simulink library "ddr4_behavioral_mdl"  (R2019b)
settings: Solver=VariableStepAuto  StartTime=0.0  StopTime=10.0  RelTol=1e-3
libraries: hdlsllib x7, simulink x4, AXIDMALib x1
settings Model: Creator=darenlee  LastModifiedBy=ajtro

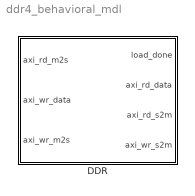
== system ddr4_behavioral_mdl ==
  DDR : Subsystem  mask{DDR3_DEPTH=1024, WR_RD_DATAWIDTH=128, INIT_DDR3=on, INIT_ADDR=0, INIT_DATA=fi(zeros(1,1024),0,128,0), OutDataTypeStr=fixdt(0,128,0), READY_DUTY_CYL=1, toggle=off}
      mask prompts: DDR3_DEPTH "DDR DEPTH"; WR_RD_DATAWIDTH "DDR Data Width"; INIT_DDR3 "Initialize DDR"; INIT_ADDR "DDR Initial Address"; INIT_DATA "DDR Initialization data"; OutDataTypeStr "Simulink:blkprm_prompts:UNIFIEDDATATYPE"; READY_DUTY_CYL "READY Duty Cycle"; toggle "Read Valid Toggling"
      mask help: DDR Simulation model
      mask init:
      | if(DDR3_DEPTH<=1)
      |     error('DDR size should be greater than 1' )  
      | end
      | 
      | if(READY_DUTY_CYL>1)
      |   error('should be less than 1' )  
      | end
      |    
      | 
      | %%Initialization Value
      | if(INIT_DDR3==true)
      |     if(isempty(INIT_ADDR))
      |      error('Enter Initial address' )  
      |     end   
      | end
      mask TypeOptions WR_RD_DATAWIDTH: 32 | 64 | 128
      mask Callback INIT_DDR3:
      | % Get the mask parameter values. This is a cell
      | %   array of character vectors.
      | maskStr = get_param(gcb,'INIT_DDR3');
      | 
      | % The pop-up menu is the first mask parameter.
      | %   Check the value selected in the pop-up
      | if strcmp(maskStr,'on')
      | 
      |     % Set the visibility of both parameters on when
      |     %   User-defined is selected in the pop-up.
      | 
      |     set_param(gcb,'MaskEnables',{'on','on','on','on','on','on','on','on'});
      | 
      | else
      | 
      |     % Turn off the visibility of the Value field
      |     %   when User-defined is not selected.
      | 
      |     set_param(gcb,'MaskEnables',{'on','on','on','off','off','on','on','on'});
      | 
      |     % Set the character vector in the Values field equal to the
      |     % character vector selected in the Gain pop-up menu.
      | 
      |     %maskStr{2}=maskStr{1};
      | 
      | end
      mask TypeOptions OutDataTypeStr: axi_wr_data/OutDataTypeStr | axi_rd_data/OutDataTypeStr
      mask DialogControl DescGroupVar Prompt: DDR
      mask DialogControl DDR3_INIT Prompt: DDR Initialization
      mask DialogControl PARAM_GROUP Prompt: DDR Initialization Parameters
      mask DialogControl OutDataTypeStr Prompt: Data type:
      mask DialogControl READY_DUTY_CYL Tooltip: between 0 to 1

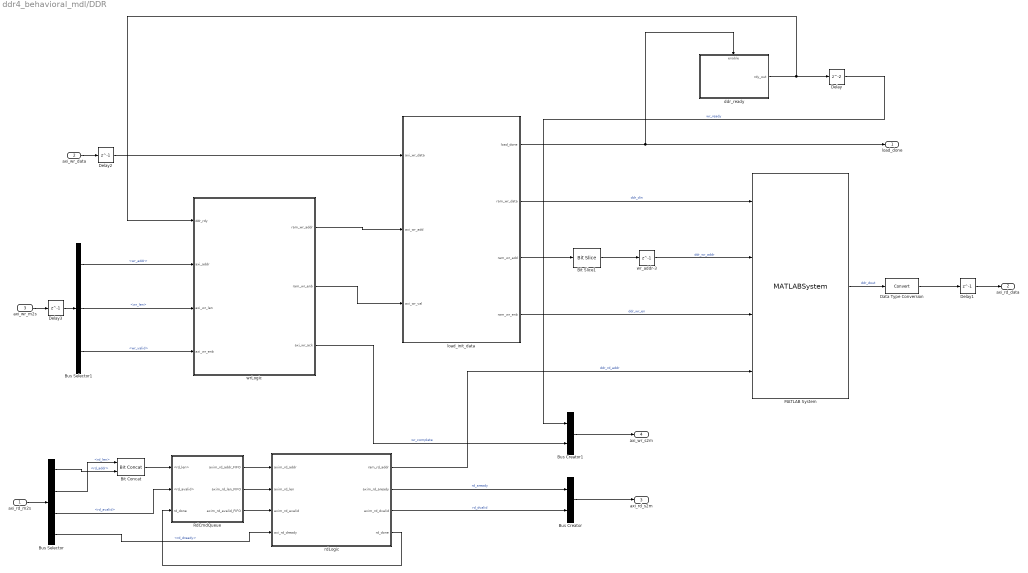
== system ddr4_behavioral_mdl/DDR ==
  axi_rd_m2s : Inport
  axi_wr_data : Inport  Port=2  OutDataTypeStr=fixdt(0,128,0)
  axi_wr_m2s : Inport  Port=3
  Bit Concat : hdlsllib/Logic and Bit Operations/Bit Concat  numInputs=2
      settings: SourceProductName=Simulink
  Bit Slice1 : hdlsllib/Logic and Bit Operations/Bit Slice  lidx=15  ridx=0
  Bus Creator : BusCreator  Inputs=2
  Bus Creator1 : BusCreator  Inputs=2
  Bus Selector : BusSelector  OutputSignals=rd_addr,rd_len,rd_avalid,rd_dready
  Bus Selector1 : BusSelector  OutputSignals=wr_addr,wr_len,wr_valid
  Data Type Conversion : DataTypeConversion
  Delay : Delay
  Delay1 : Delay  DelayLength=1
  Delay2 : Delay  DelayLength=1
  Delay3 : Delay  DelayLength=1
  MATLAB System : MATLABSystem  System=hdl.RAM  RAMType=Simple dual port  WriteOutputValue=New data  RAMInitialValue=0  SimulateUsing=Code generation
      mask Type: hdl.RAM
      mask Display:
      | disp(['Simple' char(10) 'Dual Port' char(10) 'RAM']);
      | port_label('input',1,'din');
      | port_label('input',2,'wr_addr');
      | port_label('input',3,'wr_en');
      | port_label('input',4,'rd_addr');
      | port_label('output',1,'rd_dout');
  RdCmdQueue : Subsystem
  ddr_ready : Subsystem
  load_init_data : MATLAB Function  TreatAsAtomicUnit=on
  rdLogic : Subsystem
  wrLogic : Subsystem
  wr_addr-3 : Delay  DelayLength=1
  load_done : Outport  VectorParamsAs1DForOutWhenUnconnected=off
  axi_rd_data : Outport  Port=2  OutDataTypeStr=fixdt(0,128,0)  VectorParamsAs1DForOutWhenUnconnected=off
  axi_rd_s2m : Outport  Port=3  VectorParamsAs1DForOutWhenUnconnected=off
  axi_wr_s2m : Outport  Port=4  VectorParamsAs1DForOutWhenUnconnected=off
  wires:
  Bit Slice1/1 -> wr_addr-3/1
  Delay1/1 -> axi_rd_data/1
  load_init_data/4(ram_wr_enb) -> MATLAB System/3  "ddr_wr_en"
  load_init_data/3(ram_wr_add) -> Bit Slice1/1
  load_init_data/1(load_done) -> ddr_ready/Enable, load_done/1
  MATLAB System/1 -> Data Type Conversion/1  "ddr_dout"
  rdLogic/1(ram_rd_addr) -> MATLAB System/4  "ddr_rd_addr"
  wrLogic/1(ram_wr_addr) -> load_init_data/2(axi_wr_add)
  wrLogic/2(ram_wr_enb) -> load_init_data/3(axi_wr_val)
  wr_addr-3/1 -> MATLAB System/2  "ddr_wr_addr"
  Bus Selector/1 -> Bit Concat/2  "<rd_addr>"
  Bus Selector/4 -> rdLogic/4(axi_rd_dready)  "<rd_dready>"
  axi_rd_m2s/1 -> Bus Selector/1
  Bus Selector1/1 -> wrLogic/2(axi_addr)  "<wr_addr>"
  axi_wr_m2s/1 -> Delay3/1
  Bus Selector1/3 -> wrLogic/4(axi_wr_enb)  "<wr_valid>"
  Bus Selector1/2 -> wrLogic/3(axi_wr_len)  "<wr_len>"
  rdLogic/2(axim_rd_aready) -> Bus Creator/1  "rd_aready"
  Bus Creator/1 -> axi_rd_s2m/1
  rdLogic/3(axim_rd_dvalid) -> Bus Creator/2  "rd_dvalid"
  ddr_ready/1(rdy_out) -> Delay/1, wrLogic/1(ddr_rdy)
  Bus Creator1/1 -> axi_wr_s2m/1
  wrLogic/3(axi_wr_ack) -> Bus Creator1/2  "wr_complete"
  Delay/1 -> Bus Creator1/1  "wr_ready"
  load_init_data/2(ram_wr_data) -> MATLAB System/1  "ddr_din"
  axi_wr_data/1 -> Delay2/1
  Delay2/1 -> load_init_data/1(axi_wr_data)
  Delay3/1 -> Bus Selector1/1
  Data Type Conversion/1 -> Delay1/1
  Bus Selector/2 -> Bit Concat/1  "<rd_len>"
  Bus Selector/3 -> RdCmdQueue/2(<rd_avalid>)  "<rd_avalid>"
  RdCmdQueue/2(axim_rd_len_FIFO) -> rdLogic/2(axim_rd_len)
  RdCmdQueue/3(axim_rd_avalid_FIFO) -> rdLogic/3(axim_rd_avalid)
  rdLogic/4(rd_done) -> RdCmdQueue/3(rd_done)
  Bit Concat/1 -> RdCmdQueue/1(<rd_len>)
  RdCmdQueue/1(axim_rd_addr_FIFO) -> rdLogic/1(axim_rd_addr)

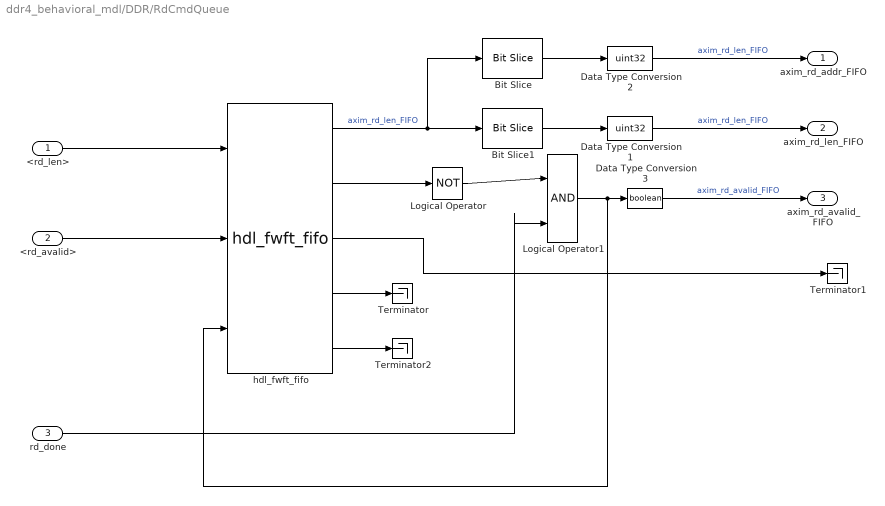
== system ddr4_behavioral_mdl/DDR/RdCmdQueue ==
  <rd_len> : Inport
  <rd_avalid> : Inport  Port=2
  rd_done : Inport  Port=3
  Bit Slice : hdlsllib/Logic and Bit Operations/Bit Slice  lidx=31  ridx=0
      settings: SourceProductName=Simulink  SourceProductBaseCode=SL
  Bit Slice1 : hdlsllib/Logic and Bit Operations/Bit Slice  lidx=63  ridx=32
      settings: SourceProductName=Simulink  SourceProductBaseCode=SL
  Data Type Conversion1 : DataTypeConversion  OutDataTypeStr=uint32
  Data Type Conversion2 : DataTypeConversion  OutDataTypeStr=uint32
  Data Type Conversion3 : DataTypeConversion  OutDataTypeStr=boolean
  Logical Operator : Logic  Operator=NOT  IconShape=distinctive  AllPortsSameDT=off  OutDataTypeStr=boolean
  Logical Operator1 : Logic  IconShape=distinctive  AllPortsSameDT=off  OutDataTypeStr=boolean
  Terminator : Terminator
  Terminator1 : Terminator
  Terminator2 : Terminator
  hdl_fwft_fifo : AXIDMALib/Hardware/hdl_fwft_fifo  FIFO_DEPTH=1*1024  AFULL_THRESH=ceil(1*1024*0.1)
  axim_rd_addr_FIFO : Outport  VectorParamsAs1DForOutWhenUnconnected=off
  axim_rd_len_FIFO : Outport  Port=2
  axim_rd_avalid_FIFO : Outport  Port=3
  wires:
  hdl_fwft_fifo/3 -> Terminator1/1
  Logical Operator1/1 -> hdl_fwft_fifo/3, Data Type Conversion3/1
  hdl_fwft_fifo/4 -> Terminator/1
  hdl_fwft_fifo/2 -> Logical Operator/1
  <rd_avalid>/1 -> hdl_fwft_fifo/2
  hdl_fwft_fifo/5 -> Terminator2/1
  Logical Operator/1 -> Logical Operator1/1
  Data Type Conversion3/1 -> axim_rd_avalid_FIFO/1  "axim_rd_avalid_FIFO"
  hdl_fwft_fifo/1 -> Bit Slice1/1, Bit Slice/1  "axim_rd_len_FIFO"
  <rd_len>/1 -> hdl_fwft_fifo/1
  rd_done/1 -> Logical Operator1/2
  Data Type Conversion1/1 -> axim_rd_len_FIFO/1  "axim_rd_len_FIFO"
  Bit Slice1/1 -> Data Type Conversion1/1
  Bit Slice/1 -> Data Type Conversion2/1
  Data Type Conversion2/1 -> axim_rd_addr_FIFO/1  "axim_rd_len_FIFO"

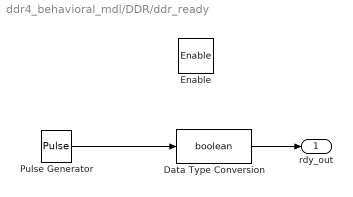
== system ddr4_behavioral_mdl/DDR/ddr_ready ==
  Enable : EnablePort
  Data Type Conversion : DataTypeConversion  OutDataTypeStr=boolean
  Pulse Generator : DiscretePulseGenerator  Period=1000  PulseWidth=1000 * READY_DUTY_CYL  SampleTime=-1
  rdy_out : Outport  VectorParamsAs1DForOutWhenUnconnected=off
  wires:
  Pulse Generator/1 -> Data Type Conversion/1
  Data Type Conversion/1 -> rdy_out/1

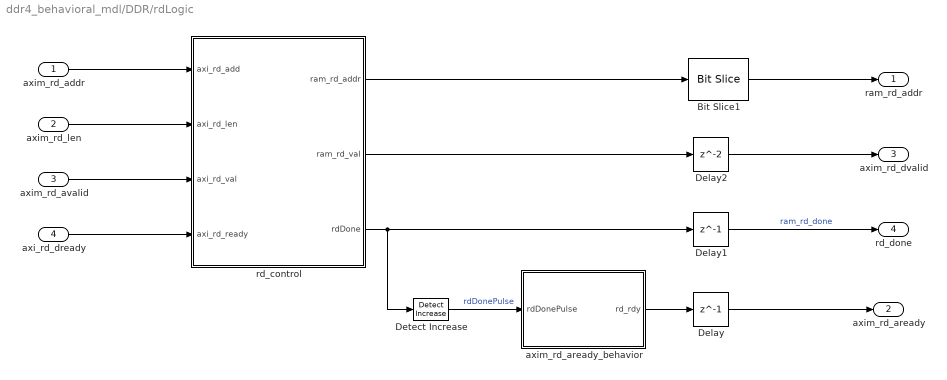
== system ddr4_behavioral_mdl/DDR/rdLogic ==
  axim_rd_addr : Inport
  axim_rd_len : Inport  Port=2
  axim_rd_avalid : Inport  Port=3
  axi_rd_dready : Inport  Port=4
  Bit Slice1 : hdlsllib/Logic and Bit Operations/Bit Slice  lidx=15  ridx=0
  Delay : Delay  DelayLength=1
  Delay1 : Delay  DelayLength=1
  Delay2 : Delay
  Detect Increase : simulink/Logic and Bit Operations/Detect Increase  vinit=0.0  OutDataTypeStr=boolean
  axim_rd_aready_behavior : MATLAB Function  TreatAsAtomicUnit=on
  rd_control : MATLAB Function  TreatAsAtomicUnit=on
  ram_rd_addr : Outport  VectorParamsAs1DForOutWhenUnconnected=off
  axim_rd_aready : Outport  Port=2  VectorParamsAs1DForOutWhenUnconnected=off
  axim_rd_dvalid : Outport  Port=3  VectorParamsAs1DForOutWhenUnconnected=off
  rd_done : Outport  Port=4  VectorParamsAs1DForOutWhenUnconnected=off
  wires:
  Delay/1 -> axim_rd_aready/1
  Detect Increase/1 -> axim_rd_aready_behavior/1(rdDonePulse)  "rdDonePulse"
  rd_control/3(rdDone) -> Delay1/1, Detect Increase/1
  axim_rd_aready_behavior/1(rd_rdy) -> Delay/1
  axim_rd_addr/1 -> rd_control/1(axi_rd_add)
  rd_control/1(ram_rd_addr) -> Bit Slice1/1
  axim_rd_avalid/1 -> rd_control/3(axi_rd_val)
  Bit Slice1/1 -> ram_rd_addr/1
  axi_rd_dready/1 -> rd_control/4(axi_rd_ready)
  Delay2/1 -> axim_rd_dvalid/1
  axim_rd_len/1 -> rd_control/2(axi_rd_len)
  rd_control/2(ram_rd_val) -> Delay2/1
  Delay1/1 -> rd_done/1  "ram_rd_done"

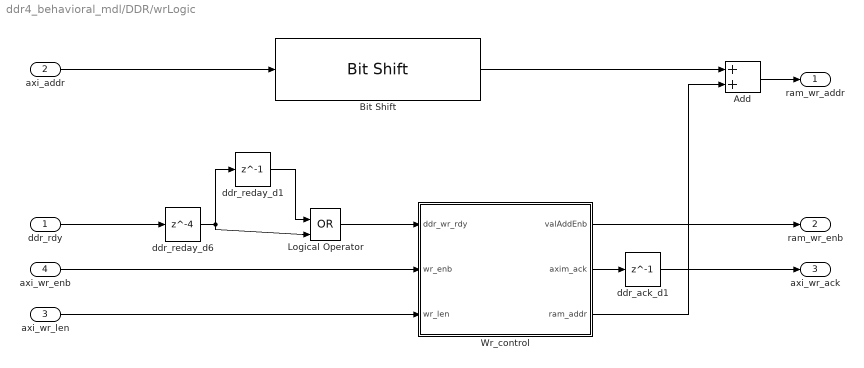
== system ddr4_behavioral_mdl/DDR/wrLogic ==
  ddr_rdy : Inport
  axi_addr : Inport  Port=2
  axi_wr_len : Inport  Port=3
  axi_wr_enb : Inport  Port=4
  Add : Sum  AccumDataTypeStr=uint32
  Bit Shift : hdlsllib/Logic and Bit Operations/Bit Shift  mode=Shift Right Arithmetic  N=log2(WR_RD_DATAWIDTH/8)
      settings: SourceProductName=HDL Coder  SourceProductBaseCode=HD
  Logical Operator : Logic  Operator=OR  IconShape=distinctive  AllPortsSameDT=off  OutDataTypeStr=boolean
  Wr_control : Subsystem
  ddr_ack_d1 : Delay  DelayLength=1
  ddr_reday_d1 : Delay  DelayLength=1
  ddr_reday_d6 : Delay  DelayLength=4
  ram_wr_addr : Outport  VectorParamsAs1DForOutWhenUnconnected=off
  ram_wr_enb : Outport  Port=2  VectorParamsAs1DForOutWhenUnconnected=off
  axi_wr_ack : Outport  Port=3  VectorParamsAs1DForOutWhenUnconnected=off
  wires:
  Wr_control/1(valAddEnb) -> ram_wr_enb/1
  axi_wr_len/1 -> Wr_control/3(wr_len)
  ddr_rdy/1 -> ddr_reday_d6/1
  axi_wr_enb/1 -> Wr_control/2(wr_enb)
  Wr_control/2(axim_ack) -> ddr_ack_d1/1
  Add/1 -> ram_wr_addr/1
  Wr_control/3(ram_addr) -> Add/2
  ddr_reday_d6/1 -> ddr_reday_d1/1, Logical Operator/2
  ddr_ack_d1/1 -> axi_wr_ack/1
  axi_addr/1 -> Bit Shift/1
  ddr_reday_d1/1 -> Logical Operator/1
  Logical Operator/1 -> Wr_control/1(ddr_wr_rdy)
  Bit Shift/1 -> Add/1

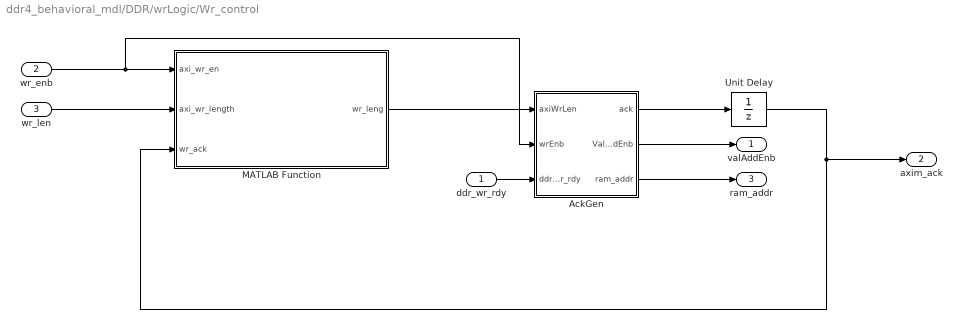
== system ddr4_behavioral_mdl/DDR/wrLogic/Wr_control ==
  ddr_wr_rdy : Inport
  wr_enb : Inport  Port=2
  wr_len : Inport  Port=3
  AckGen : Subsystem
  MATLAB Function : MATLAB Function  TreatAsAtomicUnit=on
  Unit Delay : UnitDelay  SampleTime=-1  HasFrameUpgradeWarning=on
  valAddEnb : Outport  VectorParamsAs1DForOutWhenUnconnected=off
  axim_ack : Outport  Port=2  VectorParamsAs1DForOutWhenUnconnected=off
  ram_addr : Outport  Port=3  VectorParamsAs1DForOutWhenUnconnected=off
  wires:
  wr_enb/1 -> AckGen/2(wrEnb), MATLAB Function/1(axi_wr_en)
  AckGen/2(ValAddEnb) -> valAddEnb/1
  wr_len/1 -> MATLAB Function/2(axi_wr_length)
  AckGen/1(ack) -> Unit Delay/1
  MATLAB Function/1(wr_leng) -> AckGen/1(axiWrLen)
  Unit Delay/1 -> axim_ack/1, MATLAB Function/3(wr_ack)
  AckGen/3(ram_addr) -> ram_addr/1
  ddr_wr_rdy/1 -> AckGen/3(ddr_wr_rdy)

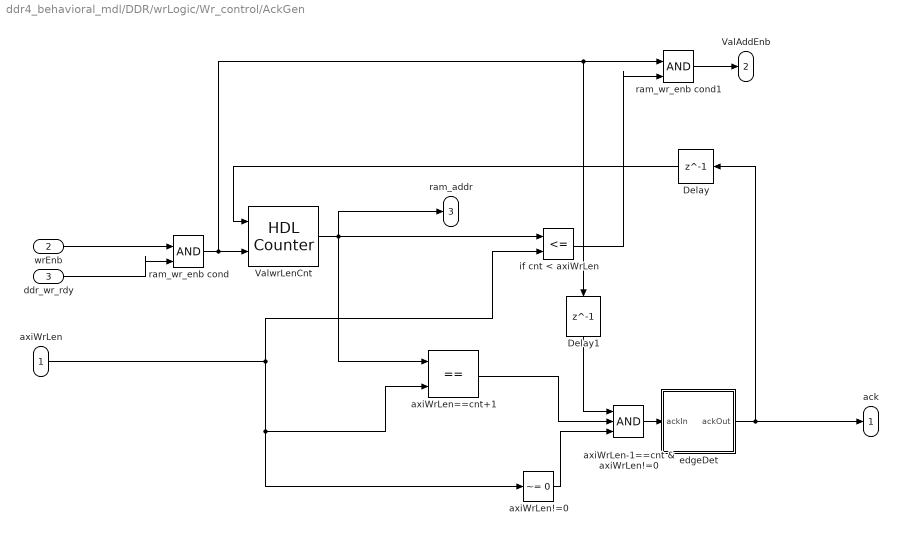
== system ddr4_behavioral_mdl/DDR/wrLogic/Wr_control/AckGen ==
  axiWrLen : Inport
  wrEnb : Inport  Port=2
  ddr_wr_rdy : Inport  Port=3
  Delay : Delay  DelayLength=1
  Delay1 : Delay  DelayLength=1
  ValwrLenCnt : hdlsllib/Sources/HDL Counter  CountType=Free running  CountInit=0  CountStep=1  CountMax=DDR3_DEPTH  CountFromType=Initial value  CountFrom=0  CountResetPort=on  CountLoadPort=off  CountEnbPort=on  CountDirPort=off  CountDataType=Unsigned  CountWordLen=32  CountFracLen=0  CountSampTime=1
      settings: SourceProductBaseCode=HD
  axiWrLen!=0 : simulink/Logic and Bit Operations/Compare To Constant  relop=~=  const=0  OutDataTypeStr=boolean
  "axiWrLen-1==cnt & axiWrLen!=0 " : Logic  Inputs=3  IconShape=distinctive  AllPortsSameDT=off  OutDataTypeStr=boolean
  axiWrLen==cnt+1 : RelationalOperator  Operator===  OutDataTypeStr=boolean  RndMeth=Nearest
  edgeDet : Subsystem
  if cnt < axiWrLen : RelationalOperator  Operator=<=  OutDataTypeStr=boolean  RndMeth=Nearest
  ram_wr_enb cond : Logic  IconShape=distinctive  AllPortsSameDT=off  OutDataTypeStr=boolean
  ram_wr_enb cond1 : Logic  IconShape=distinctive  AllPortsSameDT=off  OutDataTypeStr=boolean
  ack : Outport  VectorParamsAs1DForOutWhenUnconnected=off
  ValAddEnb : Outport  Port=2  VectorParamsAs1DForOutWhenUnconnected=off
  ram_addr : Outport  Port=3  VectorParamsAs1DForOutWhenUnconnected=off
  wires:
  "axiWrLen-1==cnt & axiWrLen!=0 "/1 -> edgeDet/1(ackIn)
  edgeDet/1(ackOut) -> ack/1, Delay/1
  axiWrLen==cnt+1/1 -> "axiWrLen-1==cnt & axiWrLen!=0 "/2
  axiWrLen!=0/1 -> "axiWrLen-1==cnt & axiWrLen!=0 "/3
  wrEnb/1 -> ram_wr_enb cond/1
  if cnt < axiWrLen/1 -> ram_wr_enb cond1/2
  axiWrLen/1 -> axiWrLen==cnt+1/2, axiWrLen!=0/1, if cnt < axiWrLen/2
  ValwrLenCnt/1 -> axiWrLen==cnt+1/1, if cnt < axiWrLen/1, ram_addr/1
  ddr_wr_rdy/1 -> ram_wr_enb cond/2
  ram_wr_enb cond/1 -> ram_wr_enb cond1/1, Delay1/1, ValwrLenCnt/2
  ram_wr_enb cond1/1 -> ValAddEnb/1
  Delay/1 -> ValwrLenCnt/1
  Delay1/1 -> "axiWrLen-1==cnt & axiWrLen!=0 "/1

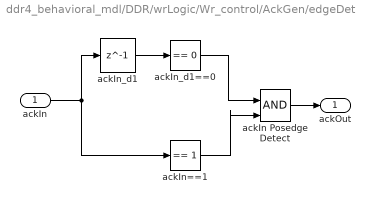
== system ddr4_behavioral_mdl/DDR/wrLogic/Wr_control/AckGen/edgeDet ==
  ackIn : Inport
  " ackIn==1" : simulink/Logic and Bit Operations/Compare To Constant  relop===  const=1  OutDataTypeStr=boolean
  ackIn Posedge Detect : Logic  IconShape=distinctive  AllPortsSameDT=off  OutDataTypeStr=boolean
  ackIn_d1 : Delay  DelayLength=1
  ackIn_d1==0 : simulink/Logic and Bit Operations/Compare To Constant  relop===  const=0  OutDataTypeStr=boolean
  ackOut : Outport  VectorParamsAs1DForOutWhenUnconnected=off
  wires:
  " ackIn==1"/1 -> ackIn Posedge Detect/2
  ackIn_d1==0/1 -> ackIn Posedge Detect/1
  ackIn Posedge Detect/1 -> ackOut/1
  ackIn_d1/1 -> ackIn_d1==0/1
  ackIn/1 -> " ackIn==1"/1, ackIn_d1/1

== matlab function ddr4_behavioral_mdl/DDR/load_init_data ==
  data: load_done output; ram_wr_data output; axi_wr_data input; axi_wr_add input; axi_wr_val input; ram_wr_add output; ram_wr_enb output boolean; INIT_ADDR parameter; DDR3_DEPTH parameter; INIT_DDR3 parameter; INIT_DATA parameter
function [load_done,ram_wr_data,ram_wr_add,ram_wr_enb] = load_init(axi_wr_data,axi_wr_add,axi_wr_val, INIT_ADDR, DDR3_DEPTH, INIT_DDR3,INIT_DATA)

%%%%%%%%%%%%%%%%%%%%%%%%%%%%%%%%%%%%%%%%%%%%%%%%%%%%%%
% Create persistent variables (registers)
persistent reg_ram_wr_add;
if(isempty(reg_ram_wr_add))
    reg_ram_wr_add = fi(0,0,32,0);
end

ram_wr_data = cast(0,'like',axi_wr_data);

persistent reg_ram_wr_data;
if(isempty(reg_ram_wr_data))
    reg_ram_wr_data =cast(0,'like',axi_wr_data);% fi(0,1,ddrWidth,0);
end

persistent reg_ram_wr_data_d1;
if(isempty(reg_ram_wr_data_d1))
    reg_ram_wr_data_d1 = cast(0,'like',axi_wr_data);%
end


persistent state;
if(isempty(state))
    state = fi(0, 0, 3, 0);
end


persistent reg_ram_wr_enb;
if(isempty(reg_ram_wr_enb))
    reg_ram_wr_enb = false;
end

persistent reg_ram_wr_enb_d1;
if(isempty(reg_ram_wr_enb_d1))
    reg_ram_wr_enb_d1 = false;
end

persistent reg_init_data;
if(isempty(reg_init_data))
    reg_init_data = cast(zeros(1,DDR3_DEPTH),'like',axi_wr_data);% fi(zeros(1,DDR3_DEPTH),1,ddrWidth,0);
end

%%%%%%%%%%%%%%%%%%%%%%%%%%%%%%%%%%%%%%%%%%%%%%%%%%
% State Memory Encoding
INIT_ST    = fi(0, 0, 3, 0);
LOAD_START = fi(1, 0, 3, 0);
LOAD_PROG  = fi(3, 0, 3, 0);
LOAD_DONE  = fi(2, 0, 3, 0);
DATA_ST    = fi(6, 0, 3, 0);


% init phase states
% 1. Every state MUST assign every output value
% 2. Use explicit data type always
switch (state)
    case INIT_ST
       
        reg_ram_wr_add = fi(0,0,32,0);%uint32(0);
        reg_ram_wr_data =  cast(0,'like',axi_wr_data);%fi(0,1,ddrWidth,0);%int32(0);
        reg_ram_wr_enb = false;
        load_done = false;
        
    case LOAD_START
        
        reg_ram_wr_add = fi(INIT_ADDR,0,32,0);
        reg_ram_wr_data =  cast(reg_init_data(1,reg_ram_wr_add+1),'like',axi_wr_data);%fi(reg_init_data(1,reg_ram_wr_add+1),1,ddrWidth,0);%int32(INIT_DATA);
        reg_ram_wr_enb = true;
        load_done = false;
    case LOAD_PROG
        
        
        reg_ram_wr_add = fi(reg_ram_wr_add+1,0,32,0);
        reg_ram_wr_data =  cast(reg_init_data(1,reg_ram_wr_add+1),'like',axi_wr_data);%fi(reg_init_data(1,reg_ram_wr_add+1),1,ddrWidth,0);%int32(INIT_DATA);
        reg_ram_wr_enb = true;
        load_done = false;
    case LOAD_DONE
      
        reg_ram_wr_add = fi(reg_ram_wr_add,0,32,0);
       % reg_ram_wr_data = reg_ram_wr_data;%fi(reg_ram_wr_data,1,ddrWidth,0);
        reg_ram_wr_enb = true;
        load_done = true;
    case DATA_ST    
        %external (AXI ) inputs
        reg_ram_wr_add = fi(axi_wr_add,0,32,0);
        reg_ram_wr_data =  axi_wr_data;%fi(axi_wr_data,1,ddrWidth,0);
        reg_ram_wr_enb = axi_wr_val;
        load_done = true;
    otherwise
        
        reg_ram_wr_add = fi(0,0,32,0);
        reg_ram_wr_data =  cast(0,'like',axi_wr_data);%fi(0,1,ddrWidth,0);
        reg_ram_wr_enb = false;
        load_done = false;
end

ram_wr_add = fi(reg_ram_wr_add,0,32,0);
%ram_wr_data = reg_ram_wr_data;

if(load_done == true)
   ram_wr_data = cast(reg_ram_wr_data_d1,'like',axi_wr_data);%fi(reg_ram_wr_data_d1,1,ddrWidth,0);%reg_ram_wr_data_d1;
else
   ram_wr_data = cast(reg_ram_wr_data_d1,'like',axi_wr_data);%fi(reg_ram_wr_data_d1,1,ddrWidth,0);%reg_ram_wr_data;   
end


if(load_done == true)
   ram_wr_enb = reg_ram_wr_enb_d1;
else
   ram_wr_enb = reg_ram_wr_enb;   
end


if(load_done == false)
   reg_init_data = cast(INIT_DATA,'like',axi_wr_data);%fi(INIT_DATA,1,ddrWidth,0);%reg_ram_wr_data;   
end

reg_ram_wr_enb_d1 = reg_ram_wr_enb;
reg_ram_wr_data_d1 = reg_ram_wr_data;%fi(reg_ram_wr_data,1,ddrWidth,0);%int32(reg_ram_wr_data);
% Next State Logic
switch (state)
    case INIT_ST
        
        if ( INIT_DDR3 == true)
            nextState = LOAD_START;
        else
            nextState = DATA_ST;
        end
    case LOAD_START
            nextState = LOAD_PROG;
    case LOAD_PROG
        if(fi(ram_wr_add,0,32,0)==fi(DDR3_DEPTH-1,0,32,0))
            nextState = LOAD_DONE;
        else
            nextState = LOAD_PROG;
        end
    case LOAD_DONE
            nextState = DATA_ST;
    case DATA_ST
            nextState = DATA_ST; 
    otherwise
        nextState = INIT_ST;
end

state = nextState;

end

== matlab function ddr4_behavioral_mdl/DDR/rdLogic/rd_control ==
  data: axi_rd_add input; axi_rd_len input; axi_rd_val input; axi_rd_ready input; ram_rd_addr output; ram_rd_val output boolean; toggle parameter; WR_RD_DATAWIDTH parameter; rdDone output
function [ram_rd_addr, ram_rd_val, rdDone] = rd_add_gen(axi_rd_add,axi_rd_len, axi_rd_val,axi_rd_ready,toggle, WR_RD_DATAWIDTH)

%%%%%%%%%%%%%%%%%%%%%%%%%%%%%%%%%%%%%%%%%%%%%%%%%%%%%%
%%%Reg declaration
%RAM address generation counter
persistent ram_rd_cnt;

RD_BYTE_STRIDE = uint32(WR_RD_DATAWIDTH/8);
rdDone = false;

if(isempty(ram_rd_cnt))
    ram_rd_cnt = fi(0,0,32,0);%uint32(0);
end

%read response ack
persistent reg_rd_ack;

if(isempty(reg_rd_ack))
    reg_rd_ack = false;
end

%read status
persistent rd_progress;

if(isempty(rd_progress))
    rd_progress = false;
end

%read addr valid flag 
persistent rd_addr_val;

if(isempty(rd_addr_val))
    rd_addr_val = false;
end

%read addr valid flag 
persistent rd_addr_val_toggle;

if(isempty(rd_addr_val_toggle))
    rd_addr_val_toggle = false;
end

%start address and length of read burst latch
persistent start_addr;
if(isempty(start_addr))
    start_addr = fi(0,0,32,0);
end

persistent leng_latch;
if(isempty(leng_latch))
    leng_latch = fi(1,0,32,0);
end

%%%%%%%%%%%%%%%%%%%%%%%%%%%%%%%%%%%%%%%%%%%%%%%
%output
ram_rd_addr = (ram_rd_cnt);
ram_rd_val = (rd_addr_val);
%%%%%%%%%%%%%%%%%%%%%%%%%%%%%%%%%%%%%%%%%%%%%%%
if((reg_rd_ack == true)&&(axi_rd_ready == true))
    ram_rd_cnt = fi(start_addr,0,32,0);%uint32(start_addr );
    rd_addr_val = true;
elseif((rd_progress == true)&&(axi_rd_ready == true))
    
    if(rd_addr_val_toggle == true)
       ram_rd_cnt = fi(ram_rd_cnt + 1,0,32,0);%uint32(ram_rd_cnt + 1);
       rd_addr_val = true;
    else
       rd_addr_val = false;
   
    end
    if(toggle)
       rd_addr_val_toggle = ~(rd_addr_val_toggle);
    else
       rd_addr_val_toggle = true;
    end
    
    TargetVal = (int32(leng_latch-1) - 1);
    if int32(ram_rd_cnt) == TargetVal
            rdDone = true;
    end
    
elseif((rd_progress == false))  
    ram_rd_cnt = fi(0,0,32,0);%uint32(0) ;
    rd_addr_val = false;
else
    rd_addr_val = false;
end


%read progress flag
if((reg_rd_ack)&&(fi(ram_rd_cnt-start_addr,0,32,0)<fi(leng_latch-1,0,32,0)))
    rd_progress = true;
elseif(fi(ram_rd_cnt-start_addr,0,32,0)==fi(leng_latch-1,0,32,0))
    rd_progress = false;
    rdDone = true; 
end


%start address , length of burst latching
if(axi_rd_val)
    leng_latch(:) = axi_rd_len;
    start_addr(:) = axi_rd_add/RD_BYTE_STRIDE;
    reg_rd_ack = true;
elseif rd_progress == false
    rdDone = true; 
    reg_rd_ack = false;
else
    reg_rd_ack = false;
end

== matlab function ddr4_behavioral_mdl/DDR/wrLogic/Wr_control/MATLAB Function ==
  data: axi_wr_en input; wr_leng output; axi_wr_length input; wr_ack input
function wr_leng = addr_latch(axi_wr_en,axi_wr_length,wr_ack)
%#codegen

persistent axi_wr_en_d1;
if(isempty(axi_wr_en_d1))
axi_wr_en_d1 = false;
end

persistent reg_len;
if(isempty(reg_len))
    reg_len = fi(0,0,32,0);%uint32(0);
end


persistent reg_len_d1;
if(isempty(reg_len_d1))
    reg_len_d1 = fi(0,0,32,0);%uint32(0);
end

reg_len_d1 = reg_len;
wr_leng = reg_len;

if((axi_wr_en==true)&&(axi_wr_en_d1==false)&&(reg_len_d1==0)) 
  reg_len= fi(axi_wr_length,0,32,0);%axi_wr_length;
elseif(wr_ack)
  reg_len= fi(0,0,32,0);%uint32(0);    
end

axi_wr_en_d1 = axi_wr_en;

== matlab function ddr4_behavioral_mdl/DDR/rdLogic/axim_rd_aready_behavior ==
  data: rdDonePulse input; rd_rdy output
function rd_rdy = aready(rdDonePulse)

persistent rdy_state delay_count
if isempty(rdy_state)
    rdy_state = uint32(0);
    delay_count = uint8(0);
end

STATE_IDLE = uint32(0);
STATE_WAIT = uint32(1);
WAIT_TIME = uint16(50);
rd_rdy = false;



switch(rdy_state)
    case(STATE_IDLE)
        if rdDonePulse % if a read just completed, wait a few moments
            rdy_state(:) = STATE_WAIT;            
        else
            rd_rdy = true;
        end
        
    case(STATE_WAIT)
        rd_rdy = false;
        
        if delay_count == WAIT_TIME
            delay_count(:) = 0;
            rdy_state(:) = STATE_IDLE;
        else
            delay_count(:) = delay_count + 1;
        end
    otherwise
        rd_rdy = false;        
end


end
